simulink model "feedforwardControl"  (R2017b)
settings: Solver=VariableStepAuto  StartTime=0.0  StopTime=37  RelTol=1e-3
undefined symbols (not defined in the file or in its folder): p560
libraries: roblocks x5
settings Model: Creator=ArsalanBangash  LastModifiedBy=ArsalanBangash

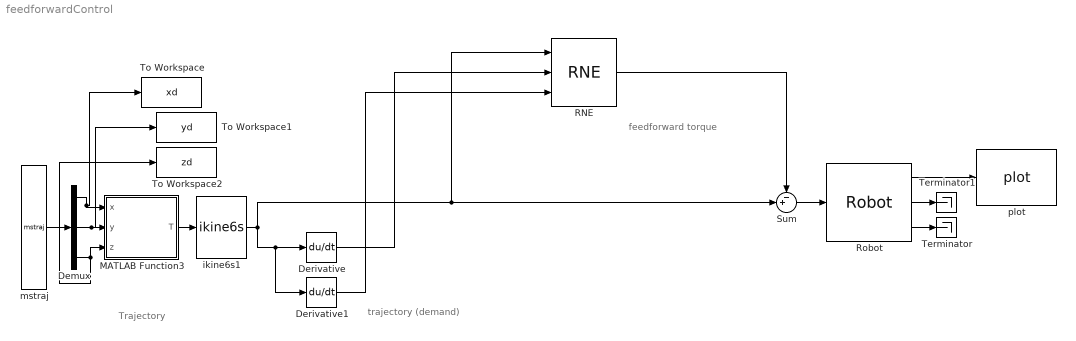
== system feedforwardControl ==
  note: feedforward torque
  note: trajectory
      | (demand)
  note: Trajectory
  Demux : Demux  Outputs=3
  Derivative : Derivative
  Derivative1 : Derivative
  MATLAB Function3 : MATLAB Function  TreatAsAtomicUnit=on
  RNE : roblocks/Arm/RNE  robot=p560.nofriction()  grav=[0 0 9.81]
  Robot : roblocks/Arm/Robot  robot=p560.nofriction  q0=[0 0 0 0 0 0]
  Sum : Sum  Inputs=-+|  SaturateOnIntegerOverflow=on  InputSameDT=on  OutDataTypeStr=Inherit: Same as first input
  Terminator : Terminator
  Terminator1 : Terminator
  To Workspace : ToWorkspace  VariableName=xd  SampleTime=-1
  To Workspace1 : ToWorkspace  VariableName=yd  SampleTime=-1
  To Workspace2 : ToWorkspace  VariableName=zd  SampleTime=-1
  ikine6s1 : roblocks/Arm/ikine6s  robot=p560  conf='luf'
  mstraj : roblocks/Toolbox/mstraj  path=|  vaxis=[0.1 0.1 0.1]  tseg=[]  dt=0.1  tacc=0  setsimtime=on
      | [ 0.5,-0.5,0.1;
      |  0.5,-0.5,0.5 ;0.5,0.5,0.5;0.5,0.5,0.1; 0.5,-0.5,0.1; 0.5,-0.5,0.5; 0.5 0 0]
  plot : roblocks/Arm/plot  robot=p560  fps=10  holdplot=on
  wires:
  Derivative/1 -> RNE/2
  Sum/1 -> Robot/1
  Robot/1 -> plot/1
  ikine6s1/1 -> Derivative1/1, Derivative/1, Sum/2, RNE/1
  Derivative1/1 -> RNE/3
  Robot/3 -> Terminator/1
  RNE/1 -> Sum/1
  Robot/2 -> Terminator1/1
  MATLAB Function3/1(T) -> ikine6s1/1
  mstraj/1 -> Demux/1
  Demux/2 -> To Workspace1/1, MATLAB Function3/2(y)
  Demux/1 -> To Workspace/1, MATLAB Function3/1(x)
  Demux/3 -> MATLAB Function3/3(z), To Workspace2/1

== matlab function feedforwardControl/MATLAB Function3 ==
  data: x input; T output; y input; z input
function T = fcn(x,y,z)

T=transl(x,y,z);
